simulink model "Test_Logic_Operations"  (Simulink 8.1)
settings: Solver=ode45  StartTime=0.0  StopTime=10.0  RelTol=1e-3
libraries: commutil2 x6, Computer_Library x4
settings Model: Creator=uzivatel  LastModifiedBy=uzivatel
settings DataIOCC: SignalLoggingSaveFormat=Dataset
settings OptimizationCC: ExpressionDepthLimit=128
settings DebuggingCC: FcnCallInpInsideContextMsg=EnableAllAsError
settings GRTTargetCC: CombineOutputUpdateFcns=on  GRTInterface=off

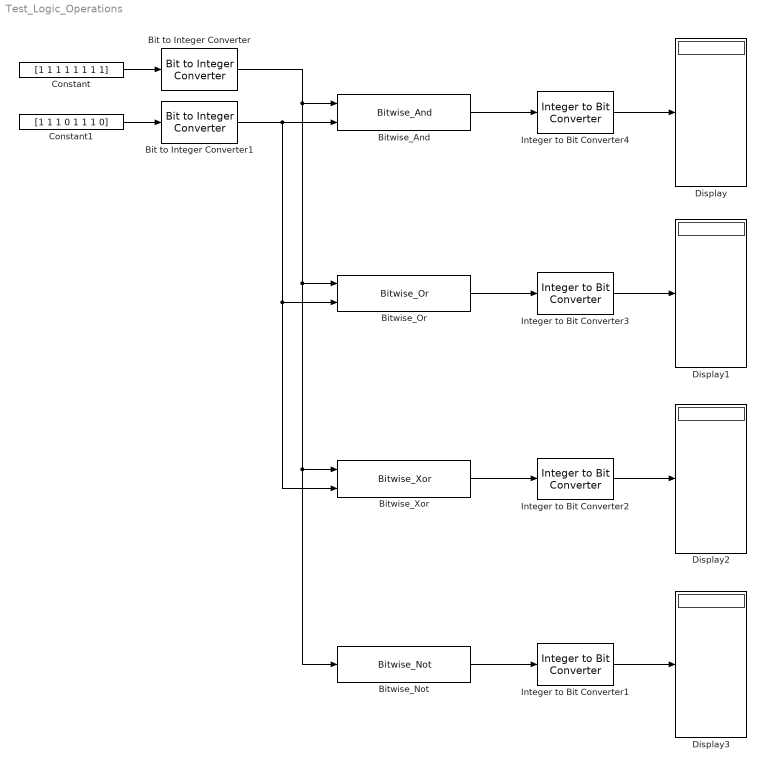
== system Test_Logic_Operations ==
  Bit to Integer Converter : commutil2/Bit to Integer Converter  nbits=8  bitOrder=MSB first  signedOutputValues=Unsigned  outDtype=uint8  outDtypeSigned=Inherit via internal rule
  Bit to Integer Converter1 : commutil2/Bit to Integer Converter  nbits=8  bitOrder=MSB first  signedOutputValues=Unsigned  outDtype=uint8  outDtypeSigned=Inherit via internal rule
  Bitwise_And : Computer_Library/Logic_Operations/Bitwise_And
  Bitwise_Not : Computer_Library/Logic_Operations/Bitwise_Not
  Bitwise_Or : Computer_Library/Logic_Operations/Bitwise_Or
  Bitwise_Xor : Computer_Library/Logic_Operations/Bitwise_Xor
  Constant : Constant  Value=[1 1 1 1 1 1 1 1]  OutDataTypeStr=uint8
  Constant1 : Constant  Value=[1 1 1 0 1 1 1 0]  OutDataTypeStr=uint8
  Display{,1..3} (4 alike) : Display
  Integer to Bit Converter{1..4} (4 alike) : commutil2/Integer to Bit Converter  nbits=8  signedInputValues=Unsigned  bitOrder=MSB first  outDtype=uint8
  wires:
  Bit to Integer Converter1/1 -> Bitwise_Xor/2, Bitwise_Or/2, Bitwise_And/2
  Bit to Integer Converter/1 -> Bitwise_Not/1, Bitwise_Xor/1, Bitwise_Or/1, Bitwise_And/1
  Bitwise_Not/1 -> Integer to Bit Converter1/1
  Integer to Bit Converter1/1 -> Display3/1
  Constant/1 -> Bit to Integer Converter/1
  Constant1/1 -> Bit to Integer Converter1/1
  Integer to Bit Converter2/1 -> Display2/1
  Bitwise_Xor/1 -> Integer to Bit Converter2/1
  Integer to Bit Converter3/1 -> Display1/1
  Bitwise_Or/1 -> Integer to Bit Converter3/1
  Integer to Bit Converter4/1 -> Display/1
  Bitwise_And/1 -> Integer to Bit Converter4/1
